simulink model "controller"  (R2020a)
settings: Solver=ode3  StartTime=0.0  StopTime=inf  FixedStep=0.01  RelTol=1e-3
libraries: robotlib x19, robotmaniplib x1
settings Model: Creator=paolo  LastModifiedBy=paolo
settings OptimizationCC: EnhancedBackFolding=on  PassReuseOutputArgsAs=Individual arguments  ZeroExternalMemoryAtStartup=off  ZeroInternalMemoryAtStartup=off  MaxStackSize=64  OptimizeBlockOrder=speed  DifferentSizesBufferReuse=on  OptimizationCustomize=off  EfficientTunableParamExpr=on
settings DebuggingCC: ParameterTunabilityLossMsg=error
settings HardwareCC: ProdBitPerPointer=32  ProdBitPerSizeT=32  ProdBitPerPtrDiffT=32  ProdLargestAtomicFloat=None  ProdIntDivRoundTo=Undefined  ProdEndianess=Unspecified  ProdWordSize=32  ProdHWDeviceType=Generic->Unspecified (assume 32-bit Generic)
settings SFSimCC: MATLABDynamicMemAlloc=off
settings RTWCC: SystemTargetFile=ert.tlc  HardwareBoard=Robot Operating System (ROS)  TemplateMakefile=ert_default_tmf  Toolchain=Catkin  TargetLang=C++
settings CodeAppCC: ForceParamTrailComments=on  IgnoreCustomStorageClasses=off  OperatorAnnotations=on  SimulinkDataObjDesc=on  SFDataObjDesc=on  InsertBlockDesc=on

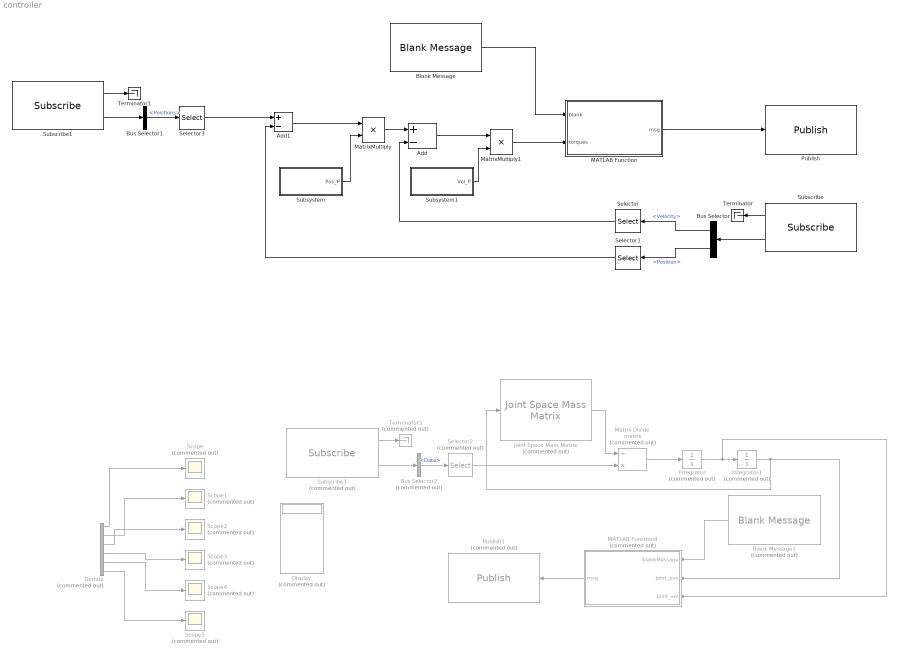
== system controller ==
  Add : Sum  Inputs=+-
  Add1 : Sum  Inputs=+-
  Blank Message : robotlib/Blank Message  messageClass=Message  entityType=std_msgs/Float64MultiArray  messageType=std_msgs/Float64MultiArray  SampleTime=inf
  Blank Message1 : robotlib/Blank Message  Commented=on  messageClass=Message  entityType=sensor_msgs/JointState  messageType=sensor_msgs/JointState  SampleTime=inf
  Bus Selector : BusSelector  OutputSignals=Velocity,Position
  Bus Selector1 : BusSelector  OutputSignals=Positions
  Bus Selector2 : BusSelector  Commented=on  OutputSignals=Data
  Demux : Demux  Commented=on  Outputs=6
  Display : Display  Commented=on
  Integrator : Integrator  Commented=on
  Integrator1 : Integrator  Commented=on
  Joint Space Mass Matrix : robotmaniplib/Joint Space Mass Matrix  Commented=on  RigidBodyTree=robot  SimulateUsing=Interpreted execution
  MATLAB Function : MATLAB Function  TreatAsAtomicUnit=on
  MATLAB Function4 : MATLAB Function  Commented=on  TreatAsAtomicUnit=on
  Matrix Divide : Product  Commented=on  Inputs=/*  Multiplication=Matrix(*)
  MatrixMultiply : Product
  MatrixMultiply1 : Product
  Publish : robotlib/Publish  topicSource=Specify your own  topic=/joint_torque  messageType=std_msgs/Float64MultiArray  messageQueueLength=1
  Publish1 : robotlib/Publish  Commented=on  topicSource=Specify your own  topic=/joint_states  messageType=sensor_msgs/JointState  messageQueueLength=1
  Scope{,1..5} (6 alike) : Scope  Commented=on
  Selector : Selector  InputPortWidth=128  IndexOptions=Starting index (dialog)  Indices=[1]  OutputSizes=6
  Selector1 : Selector  InputPortWidth=128  IndexOptions=Starting index (dialog)  Indices=1  OutputSizes=6
  Selector2 : Selector  Commented=on  IndexOptions=Starting index (dialog)  Indices=1  OutputSizes=6
  Selector3 : Selector  IndexOptions=Starting index (dialog)  Indices=1  OutputSizes=6
  Subscribe : robotlib/Subscribe  topicSource=Specify your own  topic=/joint_states  messageType=sensor_msgs/JointState  sampleTime=-1  messageQueueLength=1
  Subscribe1 : robotlib/Subscribe  topicSource=Specify your own  topic=/joint_trajectory  messageType=trajectory_msgs/JointTrajectoryPoint  sampleTime=-1  messageQueueLength=1
  Subscribe3 : robotlib/Subscribe  Commented=on  topicSource=Specify your own  topic=/joint_torque  messageType=std_msgs/Float64MultiArray  sampleTime=-1  messageQueueLength=1
  Subsystem : Subsystem
  Subsystem1 : Subsystem
  Terminator : Terminator
  Terminator1 : Terminator
  Terminator5 : Terminator  Commented=on
  wires:
  Add/1 -> MatrixMultiply1/1
  MatrixMultiply/1 -> Add/1
  MatrixMultiply1/1 -> MATLAB Function/2(torques)
  Blank Message/1 -> MATLAB Function/1(blank)
  MATLAB Function/1(msg) -> Publish/1
  Subscribe/1 -> Terminator/1
  Subscribe/2 -> Bus Selector/1
  Selector/1 -> Add/2
  Selector1/1 -> Add1/2
  Bus Selector/1 -> Selector/1  "<Velocity>"
  Bus Selector/2 -> Selector1/1  "<Position>"
  Blank Message1/1 -> MATLAB Function4/1(blankMessage)
  Selector2/1 -> Matrix Divide/2
  MATLAB Function4/1(msg) -> Publish1/1
  Subscribe3/2 -> Bus Selector2/1
  Integrator/1 -> Integrator1/1, MATLAB Function4/3(joint_vel)
  Matrix Divide/1 -> Integrator/1
  Bus Selector2/1 -> Selector2/1  "<Data>"
  Integrator1/1 -> Joint Space Mass Matrix/1, MATLAB Function4/2(joint_pos)
  Joint Space Mass Matrix/1 -> Matrix Divide/1
  Subscribe3/1 -> Terminator5/1
  Demux/2 -> Scope1/1
  Demux/3 -> Scope2/1
  Demux/4 -> Scope3/1
  Demux/5 -> Scope4/1
  Demux/6 -> Scope5/1
  Demux/1 -> Scope/1
  Add1/1 -> MatrixMultiply/1
  Subsystem/1(Pos_P) -> MatrixMultiply/2
  Subsystem1/1(Vel_P) -> MatrixMultiply1/2
  Subscribe1/1 -> Terminator1/1
  Subscribe1/2 -> Bus Selector1/1
  Selector3/1 -> Add1/1
  Bus Selector1/1 -> Selector3/1  "<Positions>"

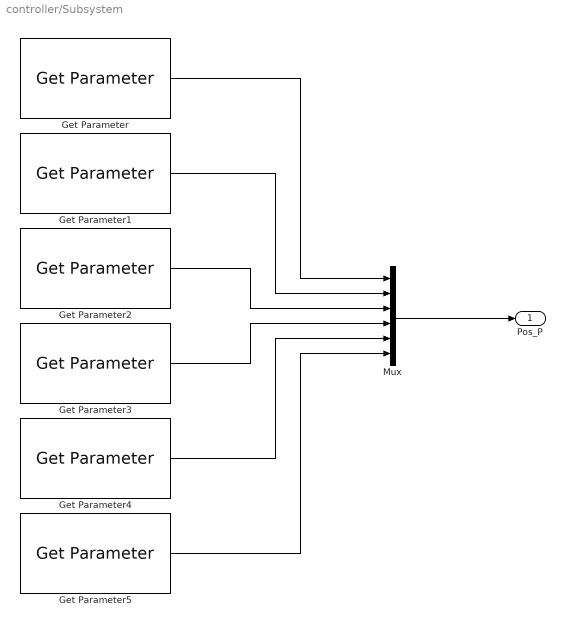
== system controller/Subsystem ==
  Get Parameter : robotlib/Get Parameter  ParameterSource=Specify your own  ParameterName=/pos_control_1  ParameterType=double  ParameterMaxArrayLength=16  ParameterInitialValue=0.2  SampleTime=-1  ShowErrorCodeOutput=off  ModelName=controller  BlockId=ParamGet_controller_93
      settings: SourceProductBaseCode=RR
  Get Parameter1 : robotlib/Get Parameter  ParameterSource=Specify your own  ParameterName=/pos_control_2  ParameterType=double  ParameterMaxArrayLength=16  ParameterInitialValue=0.2  SampleTime=-1  ShowErrorCodeOutput=off  ModelName=controller  BlockId=ParamGet_controller_94
      settings: SourceProductBaseCode=RR
  Get Parameter2 : robotlib/Get Parameter  ParameterSource=Specify your own  ParameterName=/pos_control_3  ParameterType=double  ParameterMaxArrayLength=16  ParameterInitialValue=0.2  SampleTime=-1  ShowErrorCodeOutput=off  ModelName=controller  BlockId=ParamGet_controller_95
      settings: SourceProductBaseCode=RR
  Get Parameter3 : robotlib/Get Parameter  ParameterSource=Specify your own  ParameterName=/pos_control_4  ParameterType=double  ParameterMaxArrayLength=16  ParameterInitialValue=0.2  SampleTime=-1  ShowErrorCodeOutput=off  ModelName=controller  BlockId=ParamGet_controller_96
      settings: SourceProductBaseCode=RR
  Get Parameter4 : robotlib/Get Parameter  ParameterSource=Specify your own  ParameterName=/pos_control_5  ParameterType=double  ParameterMaxArrayLength=16  ParameterInitialValue=0.2  SampleTime=-1  ShowErrorCodeOutput=off  ModelName=controller  BlockId=ParamGet_controller_97
      settings: SourceProductBaseCode=RR
  Get Parameter5 : robotlib/Get Parameter  ParameterSource=Specify your own  ParameterName=/pos_control_6  ParameterType=double  ParameterMaxArrayLength=16  ParameterInitialValue=0.2  SampleTime=-1  ShowErrorCodeOutput=off  ModelName=controller  BlockId=ParamGet_controller_98
      settings: SourceProductBaseCode=RR
  Mux : Mux  Inputs=6
  Pos_P : Outport
  wires:
  Mux/1 -> Pos_P/1
  Get Parameter/1 -> Mux/1
  Get Parameter1/1 -> Mux/2
  Get Parameter2/1 -> Mux/3
  Get Parameter3/1 -> Mux/4
  Get Parameter4/1 -> Mux/5
  Get Parameter5/1 -> Mux/6

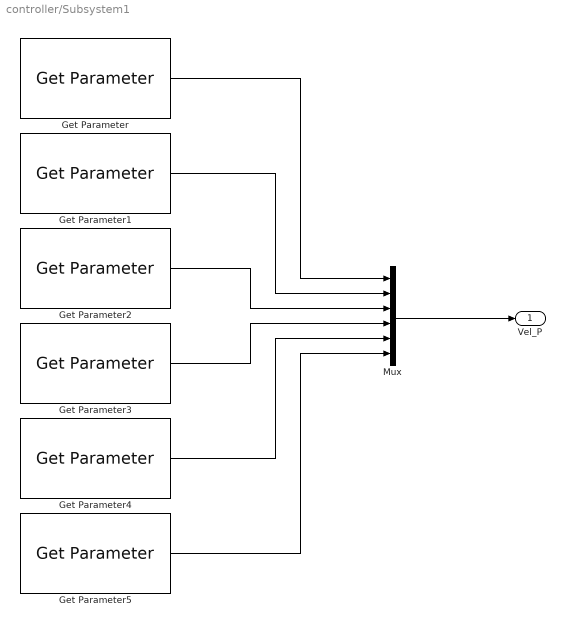
== system controller/Subsystem1 ==
  Get Parameter : robotlib/Get Parameter  ParameterSource=Specify your own  ParameterName=/vel_control_1  ParameterType=double  ParameterMaxArrayLength=16  ParameterInitialValue=0.1  SampleTime=-1  ShowErrorCodeOutput=off  ModelName=controller  BlockId=ParamGet_controller_103
      settings: SourceProductBaseCode=RR
  Get Parameter1 : robotlib/Get Parameter  ParameterSource=Specify your own  ParameterName=/vel_control_2  ParameterType=double  ParameterMaxArrayLength=16  ParameterInitialValue=0.1  SampleTime=-1  ShowErrorCodeOutput=off  ModelName=controller  BlockId=ParamGet_controller_104
      settings: SourceProductBaseCode=RR
  Get Parameter2 : robotlib/Get Parameter  ParameterSource=Specify your own  ParameterName=/vel_control_3  ParameterType=double  ParameterMaxArrayLength=16  ParameterInitialValue=0.1  SampleTime=-1  ShowErrorCodeOutput=off  ModelName=controller  BlockId=ParamGet_controller_105
      settings: SourceProductBaseCode=RR
  Get Parameter3 : robotlib/Get Parameter  ParameterSource=Specify your own  ParameterName=/vel_control_4  ParameterType=double  ParameterMaxArrayLength=16  ParameterInitialValue=0.01  SampleTime=-1  ShowErrorCodeOutput=off  ModelName=controller  BlockId=ParamGet_controller_106
      settings: SourceProductBaseCode=RR
  Get Parameter4 : robotlib/Get Parameter  ParameterSource=Specify your own  ParameterName=/vel_control_5  ParameterType=double  ParameterMaxArrayLength=16  ParameterInitialValue=0.1  SampleTime=-1  ShowErrorCodeOutput=off  ModelName=controller  BlockId=ParamGet_controller_107
      settings: SourceProductBaseCode=RR
  Get Parameter5 : robotlib/Get Parameter  ParameterSource=Specify your own  ParameterName=/vel_control_6  ParameterType=double  ParameterMaxArrayLength=16  ParameterInitialValue=1e-4  SampleTime=-1  ShowErrorCodeOutput=off  ModelName=controller  BlockId=ParamGet_controller_108
      settings: SourceProductBaseCode=RR
  Mux : Mux  Inputs=6
  Vel_P : Outport
  wires:
  Get Parameter4/1 -> Mux/5
  Mux/1 -> Vel_P/1
  Get Parameter/1 -> Mux/1
  Get Parameter5/1 -> Mux/6
  Get Parameter2/1 -> Mux/3
  Get Parameter3/1 -> Mux/4
  Get Parameter1/1 -> Mux/2

== matlab function controller/MATLAB Function4 ==
  data: blankMessage input; msg output Bus: SL_Bus_controller_joint_sensor_msgs_JointState; joint_pos input; joint_vel input
function msg = assign_message(blankMessage, joint_pos, joint_vel)

    msg = blankMessage;
    
    num_joints = length(joint_pos);
    
    msg.Position_SL_Info.CurrentLength = uint32(num_joints);
    msg.Velocity_SL_Info.CurrentLength = uint32(num_joints);
    
    for i=1:num_joints
        
        msg.Position(i) = joint_pos(i);
        msg.Velocity(i) = joint_vel(i);
        
    end

== matlab function controller/MATLAB Function ==
  data: blank input; msg output Bus: SL_Bus_controller_std_msgs_Float64MultiArray; torques input
function msg = assign_message(blank, torques)

    msg = blank;
    num_joints = length(torques);

    for i=1:num_joints
        msg.Data(i) = torques(i);
    end

    msg.Data_SL_Info.CurrentLength = uint32(num_joints);

    msg.Layout.Dim_SL_Info.CurrentLength = uint32(1);

    msg.Layout.Dim(1).Size = uint32(num_joints);
    msg.Layout.Dim(1).Stride = uint32(num_joints);
